simulink model "Feedforward"  (R2015a)
settings: Solver=ode45  StartTime=0.0  StopTime=10  RelTol=1e-3
libraries: simulink x11
PostSaveFcn:
  | % find all scope blocks as MATLAB figures:
  | set(0, 'showhiddenhandles', 'on')
  | scope = findobj(0, 'Tag', 'SIMULINK_SIMSCOPE_FIGURE');
  | for i=1:length(scope)
  |   % this is the callback of the "autoscale" button:
  |   simscope('ScopeBar', 'ActionIcon', 'Find', scope(i))
  | end
  | set(0, 'showhiddenhandles', 'off')
settings Model: Creator=Amalie  LastModifiedBy=vniel
settings DataIOCC: Refine=100

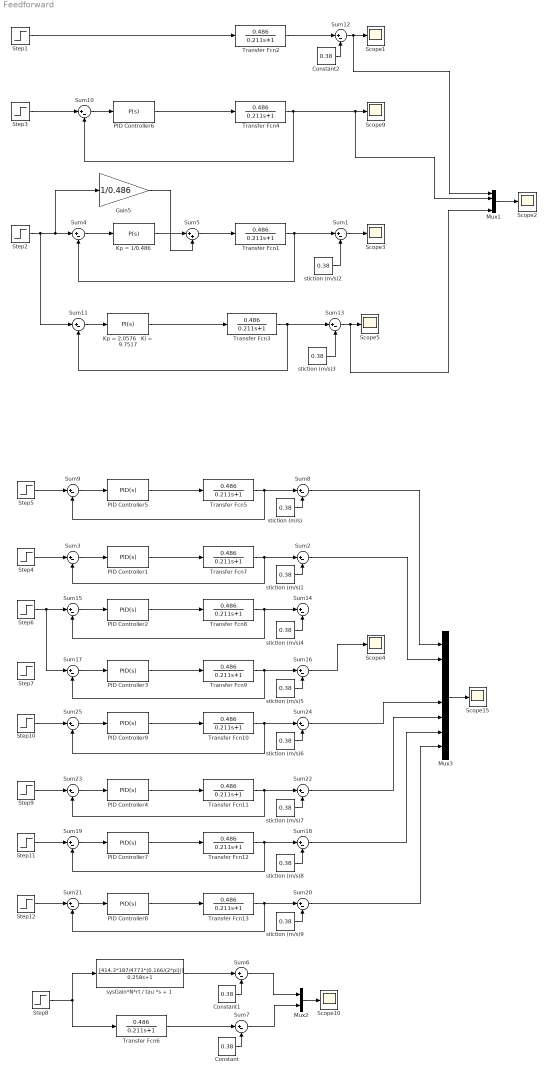
== system Feedforward ==
  Constant : Constant  Value=0.38
  Constant1 : Constant  Value=0.38
  Constant2 : Constant  Value=0.38
  Gain5 : Gain  Gain=1/0.486
  Kp = 1/0.486 : simulink/Continuous/PID Controller  Controller=P  TimeDomain=Continuous-time  SampleTime=-1  IntegratorMethod=Forward Euler  FilterMethod=Forward Euler  Form=Parallel  UseFilter=on  ControllerParametersSource=internal  P=1/0.486  I=0  D=0  N=0  InitialConditionSource=internal  InitialConditionForIntegrator=0  InitialConditionForFilter=0  ExternalReset=none  LimitOutput=off  UpperSaturationLimit=6.83  LowerSaturationLimit=0  LinearizeAsGain=on  AntiWindupMode=none  Kb=1  TrackingMode=off  Kt=1  PParamMin=[]  PParamMax=[]  IParamMin=[]  IParamMax=[]  DParamMin=[]  DParamMax=[]  NParamMin=[]  NParamMax=[]  KbParamMin=[]  KbParamMax=[]  KtParamMin=[]  KtParamMax=[]  POutMin=[]  POutMax=[]  IOutMin=[]  IOutMax=[]  DOutMin=[]  DOutMax=[]  NOutMin=[]  NOutMax=[]  KbOutMin=[]  KbOutMax=[]  KtOutMin=[]  KtOutMax=[]  IntegratorOutMin=[]  IntegratorOutMax=[]  FilterOutMin=[]  FilterOutMax=[]  SumOutMin=[]  SumOutMax=[]  SumI1OutMin=[]  SumI1OutMax=[]  SumI2OutMin=[]  SumI2OutMax=[]  SumI3OutMin=[]  SumI3OutMax=[]  SumDOutMin=[]  SumDOutMax=[]  SaturationOutMin=[]  SaturationOutMax=[]  IntegratorContinuousStateAttributes=''  IntegratorStateMustResolveToSignalObject=off  IntegratorRTWStateStorageClass=Auto  FilterContinuousStateAttributes=''  FilterStateMustResolveToSignalObject=off  FilterRTWStateStorageClass=Auto  DifferentiatorICPrevScaledInput=0  DifferentiatorOutMin=[]  DifferentiatorOutMax=[]
  Kp = 2.0576   Ki = 9.7517 : simulink/Continuous/PID Controller  Controller=PI  TimeDomain=Continuous-time  SampleTime=-1  IntegratorMethod=Forward Euler  FilterMethod=Forward Euler  Form=Parallel  UseFilter=on  ControllerParametersSource=internal  P=2.0576  I=9.7517  D=0  N=0  InitialConditionSource=internal  InitialConditionForIntegrator=0  InitialConditionForFilter=0  ExternalReset=none  LimitOutput=off  UpperSaturationLimit=7  LowerSaturationLimit=0  LinearizeAsGain=on  AntiWindupMode=none  Kb=1  TrackingMode=off  Kt=1  PParamMin=[]  PParamMax=[]  IParamMin=[]  IParamMax=[]  DParamMin=[]  DParamMax=[]  NParamMin=[]  NParamMax=[]  KbParamMin=[]  KbParamMax=[]  KtParamMin=[]  KtParamMax=[]  POutMin=[]  POutMax=[]  IOutMin=[]  IOutMax=[]  DOutMin=[]  DOutMax=[]  NOutMin=[]  NOutMax=[]  KbOutMin=[]  KbOutMax=[]  KtOutMin=[]  KtOutMax=[]  IntegratorOutMin=[]  IntegratorOutMax=[]  FilterOutMin=[]  FilterOutMax=[]  SumOutMin=[]  SumOutMax=[]  SumI1OutMin=[]  SumI1OutMax=[]  SumI2OutMin=[]  SumI2OutMax=[]  SumI3OutMin=[]  SumI3OutMax=[]  SumDOutMin=[]  SumDOutMax=[]  SaturationOutMin=[]  SaturationOutMax=[]  IntegratorContinuousStateAttributes=''  IntegratorStateMustResolveToSignalObject=off  IntegratorRTWStateStorageClass=Auto  FilterContinuousStateAttributes=''  FilterStateMustResolveToSignalObject=off  FilterRTWStateStorageClass=Auto  DifferentiatorICPrevScaledInput=0  DifferentiatorOutMin=[]  DifferentiatorOutMax=[]
  Mux1 : Mux
  Mux2 : Mux  Inputs=2
  Mux3 : Mux  Inputs=8
  PID Controller{1,3..5,7..9} (7 alike) : simulink/Continuous/PID Controller  Controller=PID  TimeDomain=Continuous-time  SampleTime=-1  IntegratorMethod=Forward Euler  FilterMethod=Forward Euler  Form=Parallel  UseFilter=on  ControllerParametersSource=internal  P=2.0576  I=9.7517  D=0  N=0  InitialConditionSource=internal  InitialConditionForIntegrator=0  InitialConditionForFilter=0  ExternalReset=none  LimitOutput=off  UpperSaturationLimit=3  LowerSaturationLimit=0  LinearizeAsGain=on  AntiWindupMode=none  Kb=1  TrackingMode=off  Kt=1  PParamMin=[]  PParamMax=[]  IParamMin=[]  IParamMax=[]  DParamMin=[]  DParamMax=[]  NParamMin=[]  NParamMax=[]  KbParamMin=[]  KbParamMax=[]  KtParamMin=[]  KtParamMax=[]  POutMin=[]  POutMax=[]  IOutMin=[]  IOutMax=[]  DOutMin=[]  DOutMax=[]  NOutMin=[]  NOutMax=[]  KbOutMin=[]  KbOutMax=[]  KtOutMin=[]  KtOutMax=[]  IntegratorOutMin=[]  IntegratorOutMax=[]  FilterOutMin=[]  FilterOutMax=[]  SumOutMin=[]  SumOutMax=[]  SumI1OutMin=[]  SumI1OutMax=[]  SumI2OutMin=[]  SumI2OutMax=[]  SumI3OutMin=[]  SumI3OutMax=[]  SumDOutMin=[]  SumDOutMax=[]  SaturationOutMin=[]  SaturationOutMax=[]  IntegratorContinuousStateAttributes=''  IntegratorStateMustResolveToSignalObject=off  IntegratorRTWStateStorageClass=Auto  FilterContinuousStateAttributes=''  FilterStateMustResolveToSignalObject=off  FilterRTWStateStorageClass=Auto  DifferentiatorICPrevScaledInput=0  DifferentiatorOutMin=[]  DifferentiatorOutMax=[]
  PID Controller2 : simulink/Continuous/PID Controller  Controller=PID  TimeDomain=Continuous-time  SampleTime=-1  IntegratorMethod=Forward Euler  FilterMethod=Forward Euler  Form=Parallel  UseFilter=on  ControllerParametersSource=internal  P=.8  I=6  D=0  N=0  InitialConditionSource=internal  InitialConditionForIntegrator=0  InitialConditionForFilter=0  ExternalReset=none  LimitOutput=off  UpperSaturationLimit=3  LowerSaturationLimit=0  LinearizeAsGain=on  AntiWindupMode=none  Kb=1  TrackingMode=off  Kt=1  PParamMin=[]  PParamMax=[]  IParamMin=[]  IParamMax=[]  DParamMin=[]  DParamMax=[]  NParamMin=[]  NParamMax=[]  KbParamMin=[]  KbParamMax=[]  KtParamMin=[]  KtParamMax=[]  POutMin=[]  POutMax=[]  IOutMin=[]  IOutMax=[]  DOutMin=[]  DOutMax=[]  NOutMin=[]  NOutMax=[]  KbOutMin=[]  KbOutMax=[]  KtOutMin=[]  KtOutMax=[]  IntegratorOutMin=[]  IntegratorOutMax=[]  FilterOutMin=[]  FilterOutMax=[]  SumOutMin=[]  SumOutMax=[]  SumI1OutMin=[]  SumI1OutMax=[]  SumI2OutMin=[]  SumI2OutMax=[]  SumI3OutMin=[]  SumI3OutMax=[]  SumDOutMin=[]  SumDOutMax=[]  SaturationOutMin=[]  SaturationOutMax=[]  IntegratorContinuousStateAttributes=''  IntegratorStateMustResolveToSignalObject=off  IntegratorRTWStateStorageClass=Auto  FilterContinuousStateAttributes=''  FilterStateMustResolveToSignalObject=off  FilterRTWStateStorageClass=Auto  DifferentiatorICPrevScaledInput=0  DifferentiatorOutMin=[]  DifferentiatorOutMax=[]
  PID Controller6 : simulink/Continuous/PID Controller  Controller=P  TimeDomain=Continuous-time  SampleTime=-1  IntegratorMethod=Forward Euler  FilterMethod=Forward Euler  Form=Parallel  UseFilter=on  ControllerParametersSource=internal  P=1/0.486  I=9.7517  D=0  N=0  InitialConditionSource=internal  InitialConditionForIntegrator=0  InitialConditionForFilter=0  ExternalReset=none  LimitOutput=off  UpperSaturationLimit=3  LowerSaturationLimit=0  LinearizeAsGain=on  AntiWindupMode=none  Kb=1  TrackingMode=off  Kt=1  PParamMin=[]  PParamMax=[]  IParamMin=[]  IParamMax=[]  DParamMin=[]  DParamMax=[]  NParamMin=[]  NParamMax=[]  KbParamMin=[]  KbParamMax=[]  KtParamMin=[]  KtParamMax=[]  POutMin=[]  POutMax=[]  IOutMin=[]  IOutMax=[]  DOutMin=[]  DOutMax=[]  NOutMin=[]  NOutMax=[]  KbOutMin=[]  KbOutMax=[]  KtOutMin=[]  KtOutMax=[]  IntegratorOutMin=[]  IntegratorOutMax=[]  FilterOutMin=[]  FilterOutMax=[]  SumOutMin=[]  SumOutMax=[]  SumI1OutMin=[]  SumI1OutMax=[]  SumI2OutMin=[]  SumI2OutMax=[]  SumI3OutMin=[]  SumI3OutMax=[]  SumDOutMin=[]  SumDOutMax=[]  SaturationOutMin=[]  SaturationOutMax=[]  IntegratorContinuousStateAttributes=''  IntegratorStateMustResolveToSignalObject=off  IntegratorRTWStateStorageClass=Auto  FilterContinuousStateAttributes=''  FilterStateMustResolveToSignalObject=off  FilterRTWStateStorageClass=Auto  DifferentiatorICPrevScaledInput=0  DifferentiatorOutMin=[]  DifferentiatorOutMax=[]
  Scope{1..5,9..10,15} (8 alike) : Scope
      Scope1 settings: TimeRange=10  YMin=-1  YMax=1
      Scope10 settings: TimeRange=10  YMin=-1  YMax=1  SaveName=ScopeData8
      Scope15 settings: TimeRange=10  SaveName=ScopeData14
      Scope2 settings: TimeRange=10  YMin=-0.4  YMax=0
      Scope3 settings: TimeRange=10  SaveName=ScopeData3
      Scope4 settings: TimeRange=10  SaveName=ScopeData4
      Scope5 settings: TimeRange=10  SaveName=ScopeData2
      Scope9 settings: TimeRange=10  SaveName=ScopeData7
  Step1 : Step  Time=3  Before=0.38/0.486  After=1.4/0.486+0.38/0.486  SampleTime=0
  Step10 : Step  Time=3  Before=0.3+0.38  After=1.8+0.38  SampleTime=0
  Step11 : Step  Time=3  Before=0.3+0.38  After=2.2+0.38  SampleTime=0
  Step12 : Step  Time=3  Before=0.3+0.38  After=2.4+0.38  SampleTime=0
  Step2 : Step  Time=3  Before=0.232+0.38  After=1.4+0.38  SampleTime=0
  Step3 : Step  Time=3  After=1.4  SampleTime=0
  Step4 : Step  Time=3  Before=0.3+0.38  After=1.2+0.38  SampleTime=0
  Step5 : Step  Time=3  Before=0.3+0.38  After=1+0.38  SampleTime=0
  Step6 : Step  Time=3  Before=0.21+0.38  After=1.4+0.38  SampleTime=0
  Step7 : Step  Time=3  Before=0.3+0.38  After=1.6+0.38  SampleTime=0
  Step8 : Step  Time=2  After=7  SampleTime=0
  Step9 : Step  Time=3  Before=0.3+0.38  After=2+0.38  SampleTime=0
  Sum{1..4,6..25} (24 alike) : Sum  Inputs=|+-
  Sum5 : Sum  Inputs=|++
  Transfer Fcn{1..13} (13 alike) : TransferFcn  Numerator=[0.486]  Denominator=[0.211 1]
  stiction (m/s){,1..9} (10 alike) : Constant  Value=0.38
  sysGain*N*rt / tau *s + 1 : TransferFcn  Numerator=[414.3*187/4773*(0.166/(2*pi))]  Denominator=[0.258 1]
  wires:
  Sum4/1 -> Kp = 1/0.486/1
  Sum5/1 -> Transfer Fcn1/1
  Kp = 1/0.486/1 -> Sum5/1
  Mux1/1 -> Scope2/1
  Step5/1 -> Sum9/1
  Transfer Fcn5/1 -> Sum8/1, Sum9/2
  Transfer Fcn6/1 -> Sum7/1
  Mux2/1 -> Scope10/1
  Constant/1 -> Sum7/2
  Sum7/1 -> Mux2/2
  Step8/1 -> Transfer Fcn6/1, sysGain*N*rt / tau *s + 1/1
  stiction (m/s)/1 -> Sum8/2
  Constant1/1 -> Sum6/2
  Sum6/1 -> Mux2/1
  sysGain*N*rt / tau *s + 1/1 -> Sum6/1
  Sum9/1 -> PID Controller5/1
  PID Controller5/1 -> Transfer Fcn5/1
  Transfer Fcn4/1 -> Mux1/2, Scope9/1, Sum10/2
  Sum10/1 -> PID Controller6/1
  Transfer Fcn1/1 -> Sum1/1, Sum4/2
  stiction (m/s)2/1 -> Sum1/2
  Sum1/1 -> Scope3/1
  Transfer Fcn2/1 -> Sum12/1
  Constant2/1 -> Sum12/2
  Sum12/1 -> Mux1/1, Scope1/1
  Transfer Fcn3/1 -> Sum13/1, Sum11/2
  Sum13/1 -> Mux1/4, Scope5/1
  stiction (m/s)3/1 -> Sum13/2
  Sum11/1 -> Kp = 2.0576   Ki = 9.7517/1
  Kp = 2.0576   Ki = 9.7517/1 -> Transfer Fcn3/1
  Step1/1 -> Transfer Fcn2/1
  PID Controller6/1 -> Transfer Fcn4/1
  Step2/1 -> Sum11/1, Gain5/1, Sum4/1
  Gain5/1 -> Sum5/2
  Step3/1 -> Sum10/1
  Step4/1 -> Sum3/1
  Transfer Fcn7/1 -> Sum3/2, Sum2/1
  stiction (m/s)1/1 -> Sum2/2
  Sum3/1 -> PID Controller1/1
  PID Controller1/1 -> Transfer Fcn7/1
  Transfer Fcn8/1 -> Sum14/1, Sum15/2
  stiction (m/s)4/1 -> Sum14/2
  Sum15/1 -> PID Controller2/1
  PID Controller2/1 -> Transfer Fcn8/1
  Transfer Fcn9/1 -> Sum17/2, Sum16/1
  stiction (m/s)5/1 -> Sum16/2
  Sum17/1 -> PID Controller3/1
  PID Controller3/1 -> Transfer Fcn9/1
  Step10/1 -> Sum25/1
  Transfer Fcn10/1 -> Sum25/2, Sum24/1
  stiction (m/s)6/1 -> Sum24/2
  Sum25/1 -> PID Controller9/1
  PID Controller9/1 -> Transfer Fcn10/1
  Step9/1 -> Sum23/1
  Transfer Fcn11/1 -> Sum22/1, Sum23/2
  stiction (m/s)7/1 -> Sum22/2
  Sum23/1 -> PID Controller4/1
  PID Controller4/1 -> Transfer Fcn11/1
  Step11/1 -> Sum19/1
  Transfer Fcn12/1 -> Sum19/2, Sum18/1
  stiction (m/s)8/1 -> Sum18/2
  Sum19/1 -> PID Controller7/1
  PID Controller7/1 -> Transfer Fcn12/1
  Step12/1 -> Sum21/1
  Transfer Fcn13/1 -> Sum20/1, Sum21/2
  stiction (m/s)9/1 -> Sum20/2
  Sum21/1 -> PID Controller8/1
  PID Controller8/1 -> Transfer Fcn13/1
  Mux3/1 -> Scope15/1
  Sum8/1 -> Mux3/1
  Sum20/1 -> Mux3/8
  Sum18/1 -> Mux3/7
  Sum22/1 -> Mux3/6
  Sum24/1 -> Mux3/5
  Sum2/1 -> Mux3/2
  Step6/1 -> Sum17/1, Sum15/1
  Sum16/1 -> Scope4/1
